simulink model "Closedloop"  (R2015b)
settings: Solver=ode4  StartTime=0.0  StopTime=600  FixedStep=DT  MaxStep=DT  RelTol=1e-3
values from neighbouring files (symbols this model uses):
  A1 = 1/Jr    (= 3.37837837838e-07)    [Run_closedloop.m]    (also in Run_img_closedloop.m)
  A2 = (Jr*(lambda-b31)-Cr)/Jr^2    [Run_closedloop.m]    (also in Run_img_closedloop.m)
  A3 = (Cr^2-a31*Jr-lambda*Cr*Jr)/Jr^2    [Run_closedloop.m]    (also in Run_img_closedloop.m)
  A4 = -a32/Jr    (= 0.00215037048063)    [Run_closedloop.m]    (also in Run_img_closedloop.m)
  A5 = (Cr-a33*Jr-lambda*Jr)/Jr^2    [Run_closedloop.m]    (also in Run_img_closedloop.m)
  b32 = Cls/ng/Jg    (= 21.4347948375)    [Run_closedloop.m]    (also in Run_img_closedloop.m)
  beta_opt = 2    [Run_closedloop.m]    (also in Run_img_closedloop.m)
  Cp = xlsread(filename)    [Run_closedloop.m]    (also in Run_img_closedloop.m)
  Cr = 625    [Run_closedloop.m]    (also in Run_img_closedloop.m)
  eta = 0.01    [Run_closedloop.m]    (also in Run_img_closedloop.m = 0.05)
  Jr = 2.96e6    (= 2960000)    [Run_closedloop.m]    (also in Run_img_closedloop.m)
  lambda = 0.1    [Run_closedloop.m]    (also in Run_img_closedloop.m = 10)
  lambda_opt = 7.1    [Run_closedloop.m]    (also in Run_img_closedloop.m)
  phi = 0.1    [Run_closedloop.m]    (also in Run_img_closedloop.m = 0.001)
  R = 35    [Run_closedloop.m]    (also in Run_img_closedloop.m)
  Rho = 1.225    [Run_closedloop.m]    (also in Run_img_closedloop.m)
undefined symbols (not defined in the file or in its folder): OutList, strmatch
settings Model: Creator=bjonkman  LastModifiedBy=alino
settings DataIOCC: SaveFormat=Array  SignalLoggingSaveFormat=ModelDataLogs  SaveOutput=off  SaveTime=off  SignalLoggingName=sigsOut
settings OptimizationCC: ExpressionDepthLimit=2147483647
settings DebuggingCC: SaveWithParameterizedLinksMsg=none  UnderspecifiedInitializationDetection=Classic  MergeDetectMultiDrivingBlocksExec=none  SignalResolutionControl=TryResolveAllWithWarning  MultiTaskDSMMsg=warning  MultiTaskCondExecSysMsg=none  FcnCallInpInsideContextMsg=EnableAllAsWarning  StateNameClashWarn=warning
settings HardwareCC: ProdBitPerPointer=32  ProdLargestAtomicFloat=None  ProdIntDivRoundTo=Undefined  ProdEndianess=Unspecified  ProdWordSize=32  ProdHWDeviceType=32-bit Generic  TargetUnknown=on
settings GRTTargetCC: GeneratePreprocessorConditionals=Disable all  CombineOutputUpdateFcns=off  GRTInterface=on
settings ConfigComp: CovModelRefEnable=Off

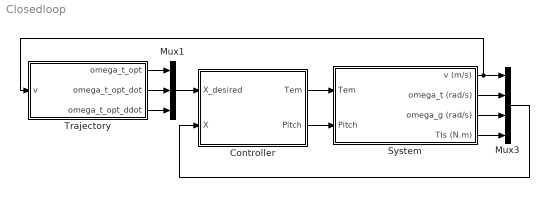
== system Closedloop ==
  Controller : Subsystem
  Mux1 : Mux  Inputs=3
  Mux3 : Mux
  System : Subsystem
  Trajectory : Subsystem
  wires:
  Mux3/1 -> Controller/2(X)
  Mux1/1 -> Controller/1(X_desired)
  Trajectory/2(omega_t_opt_dot) -> Mux1/2
  Trajectory/1(omega_t_opt) -> Mux1/1
  Controller/1(Tem) -> System/1(Tem)
  Controller/2(Pitch) -> System/2(Pitch)
  System/3(omega_g (rad/s)) -> Mux3/3
  System/4(Tls (N.m)) -> Mux3/4
  System/2(omega_t (rad/s)) -> Mux3/2
  System/1(v (m/s)) -> Mux3/1, Trajectory/1(v)
  Trajectory/3(omega_t_opt_ddot) -> Mux1/3

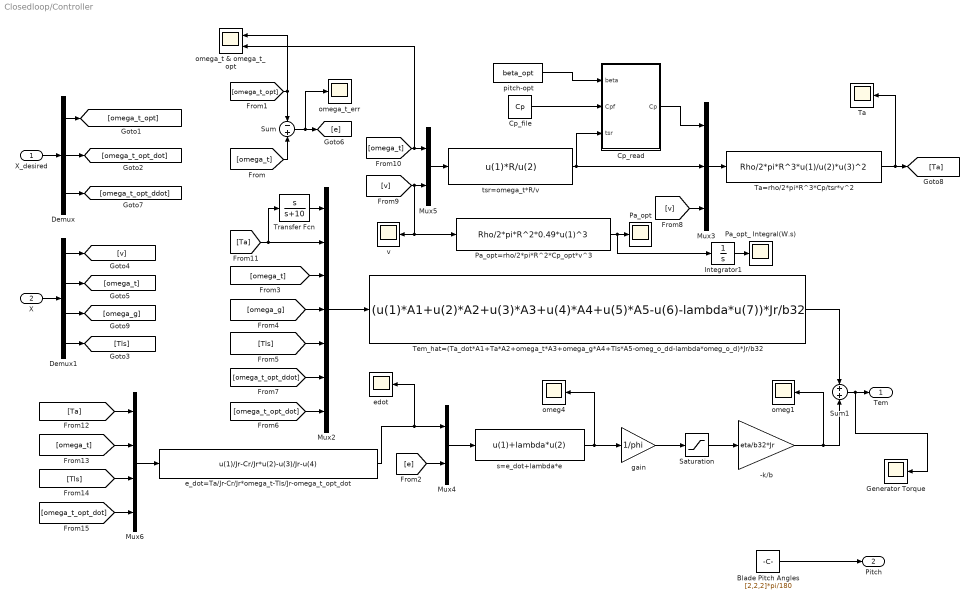
== system Closedloop/Controller ==
  X_desired : Inport
  X : Inport  Port=2
  -k/b : Gain  Gain=eta/b32*Jr
  Blade Pitch Angles : Constant  Value=[2,2,2]*pi/180
  Cp_file : Constant  Value=Cp
  Cp_read : MATLAB Function  TreatAsAtomicUnit=on
  Demux : Demux  Outputs=3
  Demux1 : Demux
  Generator Torque : Scope
  Integrator1 : Integrator
  Mux2 : Mux  Inputs=7
  Mux3 : Mux  Inputs=3
  Mux4 : Mux  Inputs=2
  Mux5 : Mux  Inputs=2
  Mux6 : Mux
  Pa_opt : Scope
  Pa_opt=rho/2*pi*R^2*Cp_opt*v^3 : Fcn  Expr=Rho/2*pi*R^2*0.49*u(1)^3
  Pa_opt_ Integral(W.s) : Scope
  Saturation : Saturate  UpperLimit=1  LowerLimit=-1
  Sum : Sum  Inputs=-+
  Sum1 : Sum  Inputs=+|+
  Ta : Scope
  Ta=rho/2*pi*R^3*Cp/tsr*v^2 : Fcn  Expr=Rho/2*pi*R^3*u(1)/u(2)*u(3)^2
  Tem_hat=(Ta_dot*A1+Ta*A2+omega_t*A3+omega_g*A4+Tls*A5-omeg_o_dd-lambda*omeg_o_d)*Jr/b32 : Fcn  Expr=(u(1)*A1+u(2)*A2+u(3)*A3+u(4)*A4+u(5)*A5-u(6)-lambda*u(7))*Jr/b32
  Transfer Fcn : TransferFcn  Numerator=[1 0]  Denominator=[1 10]
  e_dot=Ta/Jr-Cr/Jr*omega_t-Tls/Jr-omega_t_opt_dot : Fcn  Expr=u(1)/Jr-Cr/Jr*u(2)-u(3)/Jr-u(4)
  edot : Scope
  gain : Gain  Gain=1/phi
  omeg1 : Scope
  omeg4 : Scope
  omega_t & omega_t_opt : Scope  NumInputPorts=2
  omega_t_err : Scope
  pitch-opt : Constant  Value=beta_opt
  s=e_dot+lambda*e : Fcn  Expr=u(1)+lambda*u(2)
  tsr=omega_t*R/v : Fcn  Expr=u(1)*R/u(2)
  v : Scope
  Tem : Outport
  Pitch : Outport  Port=2
  wires:
  X_desired/1 -> Demux/1
  X/1 -> Demux1/1
  Tem_hat=(Ta_dot*A1+Ta*A2+omega_t*A3+omega_g*A4+Tls*A5-omeg_o_dd-lambda*omeg_o_d)*Jr/b32/1 -> Sum1/1
  Mux2/1 -> Tem_hat=(Ta_dot*A1+Ta*A2+omega_t*A3+omega_g*A4+Tls*A5-omeg_o_dd-lambda*omeg_o_d)*Jr/b32/1
  Mux4/1 -> s=e_dot+lambda*e/1
  s=e_dot+lambda*e/1 -> gain/1, omeg4/1
  [omega_t] -> Mux2/3
  Demux/1 -> [omega_t_opt]
  Demux/2 -> [omega_t_opt_dot]
  Demux1/1 -> [v]
  Demux1/2 -> [omega_t]
  Demux1/3 -> [omega_g]
  Blade Pitch Angles/1 -> Pitch/1
  Demux1/4 -> [Tls]
  Sum/1 -> omega_t_err/1, [e]
  [omega_t] -> Sum/2
  [omega_t_opt] -> omega_t & omega_t_opt/1, Sum/1
  [e] -> Mux4/2
  Demux/3 -> [omega_t_opt_ddot]
  [omega_g] -> Mux2/4
  [Tls] -> Mux2/5
  Mux3/1 -> Ta=rho/2*pi*R^3*Cp/tsr*v^2/1
  [v] -> Mux3/3
  Mux5/1 -> tsr=omega_t*R/v/1
  [v] -> Pa_opt=rho/2*pi*R^2*Cp_opt*v^3/1, v/1, Mux5/2
  [omega_t] -> omega_t & omega_t_opt/2, Mux5/1
  tsr=omega_t*R/v/1 -> Mux3/2, Cp_read/3(tsr)
  Ta=rho/2*pi*R^3*Cp/tsr*v^2/1 -> Ta/1, [Ta]
  [Ta] -> Transfer Fcn/1, Mux2/2
  Transfer Fcn/1 -> Mux2/1
  Mux6/1 -> e_dot=Ta/Jr-Cr/Jr*omega_t-Tls/Jr-omega_t_opt_dot/1
  e_dot=Ta/Jr-Cr/Jr*omega_t-Tls/Jr-omega_t_opt_dot/1 -> edot/1, Mux4/1
  [Ta] -> Mux6/1
  [omega_t] -> Mux6/2
  [Tls] -> Mux6/3
  [omega_t_opt_dot] -> Mux6/4
  Cp_read/1(Cp) -> Mux3/1
  Cp_file/1 -> Cp_read/2(Cpf)
  pitch-opt/1 -> Cp_read/1(beta)
  Sum1/1 -> Generator Torque/1, Tem/1
  [omega_t_opt_dot] -> Mux2/7
  [omega_t_opt_ddot] -> Mux2/6
  Saturation/1 -> -k/b/1
  gain/1 -> Saturation/1
  -k/b/1 -> omeg1/1, Sum1/2
  Pa_opt=rho/2*pi*R^2*Cp_opt*v^3/1 -> Integrator1/1, Pa_opt/1
  Integrator1/1 -> Pa_opt_ Integral(W.s)/1

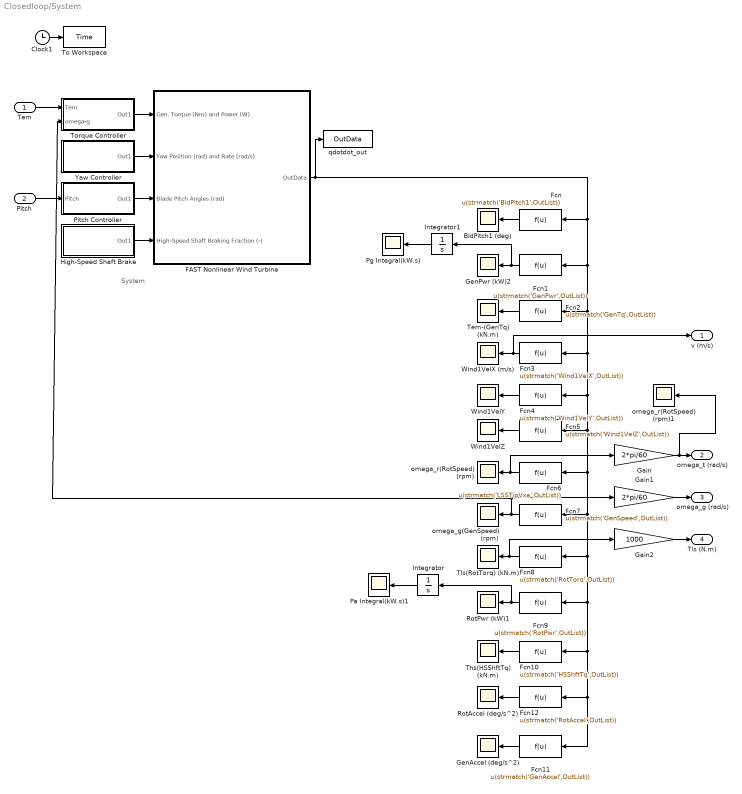
== system Closedloop/System ==
  note: System
  Tem : Inport
  Pitch : Inport  Port=2
  BldPitch1 (deg) : Scope
  Clock1 : Clock
  FAST Nonlinear Wind Turbine : Subsystem  mask(FAST Nonlinear Wind Turbine){}
      mask help: This block contains the FAST S-Function.
      mask init:
      | clear FAST_SFunc
  Fcn : Fcn  Expr=u(strmatch('BldPitch1',OutList))
  Fcn1 : Fcn  Expr=u(strmatch('GenPwr',OutList))
  Fcn10 : Fcn  Expr=u(strmatch('HSShftTq',OutList))
  Fcn11 : Fcn  Expr=u(strmatch('GenAccel',OutList))
  Fcn12 : Fcn  Expr=u(strmatch('RotAccel',OutList))
  Fcn2 : Fcn  Expr=u(strmatch('GenTq',OutList))
  Fcn3 : Fcn  Expr=u(strmatch('Wind1VelX',OutList))
  Fcn4 : Fcn  Expr=u(strmatch('Wind1VelY',OutList))
  Fcn5 : Fcn  Expr=u(strmatch('Wind1VelZ',OutList))
  Fcn6 : Fcn  Expr=u(strmatch('LSSTipVxa',OutList))
  Fcn7 : Fcn  Expr=u(strmatch('GenSpeed',OutList))
  Fcn8 : Fcn  Expr=u(strmatch('RotTorq',OutList))
  Fcn9 : Fcn  Expr=u(strmatch('RotPwr',OutList))
  Gain : Gain  Gain=2*pi/60
  Gain1 : Gain  Gain=2*pi/60
  Gain2 : Gain  Gain=1000
  GenAccel (deg/s^2) : Scope
  GenPwr (kW)2 : Scope
  High-Speed Shaft Brake : Subsystem
  Integrator : Integrator
  Integrator1 : Integrator
  Pa Integral(kW.s)1 : Scope
  Pg Integral(kW.s) : Scope
  Pitch Controller : Subsystem
  RotAccel (deg/s^2) : Scope
  RotPwr (kW)1 : Scope
  Tem-(GenTq) (kN.m) : Scope
  Ths(HSShftTq) (kN.m) : Scope
  Tls(RotTorq) (kN.m) : Scope
  To Workspace : ToWorkspace  VariableName=Time  SampleTime=-1
  Torque Controller : Subsystem
  Wind1VelX (m/s) : Scope
  Wind1VelY : Scope
  Wind1VelZ : Scope
  Yaw Controller : Subsystem
  omega_g(GenSpeed) (rpm) : Scope
  omega_r(RotSpeed) (rpm) : Scope
  omega_r(RotSpeed) (rpm)1 : Scope
  qdotdot_out : ToWorkspace  VariableName=OutData  SampleTime=-1
  v (m/s) : Outport
  omega_t (rad/s) : Outport  Port=2
  omega_g (rad/s) : Outport  Port=3
  Tls (N.m) : Outport  Port=4
  wires:
  Clock1/1 -> To Workspace/1
  Torque Controller/1(Out1) -> FAST Nonlinear Wind Turbine/1(Gen. Torque (Nm) and Power (W))
  Yaw Controller/1(Out1) -> FAST Nonlinear Wind Turbine/2(Yaw Position (rad) and Rate (rad/s))
  Pitch Controller/1(Out1) -> FAST Nonlinear Wind Turbine/3(Blade Pitch Angles (rad))
  High-Speed Shaft Brake/1(Out1) -> FAST Nonlinear Wind Turbine/4(High-Speed Shaft Braking Fraction (-))
  Fcn/1 -> BldPitch1 (deg)/1
  Fcn2/1 -> Tem-(GenTq) (kN.m)/1
  Fcn3/1 -> v (m/s)/1, Wind1VelX (m/s)/1
  Fcn4/1 -> Wind1VelY/1
  Fcn5/1 -> Wind1VelZ/1
  Fcn6/1 -> Gain/1, omega_r(RotSpeed) (rpm)/1
  Fcn7/1 -> Torque Controller/2(omega-g), Gain1/1, omega_g(GenSpeed) (rpm)/1
  Fcn8/1 -> Gain2/1, Tls(RotTorq) (kN.m)/1
  Fcn9/1 -> RotPwr (kW)1/1, Integrator/1
  Fcn10/1 -> Ths(HSShftTq) (kN.m)/1
  Fcn12/1 -> RotAccel (deg/s^2)/1
  FAST Nonlinear Wind Turbine/1(OutData) -> Fcn11/1, Fcn12/1, Fcn10/1, Fcn9/1, Fcn8/1, Fcn7/1, Fcn6/1, Fcn5/1, Fcn4/1, Fcn3/1, Fcn2/1, Fcn1/1, Fcn/1, qdotdot_out/1
  Fcn11/1 -> GenAccel (deg/s^2)/1
  Tem/1 -> Torque Controller/1(Tem)
  Gain/1 -> omega_r(RotSpeed) (rpm)1/1, omega_t (rad/s)/1
  Gain1/1 -> omega_g (rad/s)/1
  Gain2/1 -> Tls (N.m)/1
  Pitch/1 -> Pitch Controller/1(Pitch)
  Integrator/1 -> Pa Integral(kW.s)1/1
  Fcn1/1 -> GenPwr (kW)2/1, Integrator1/1
  Integrator1/1 -> Pg Integral(kW.s)/1

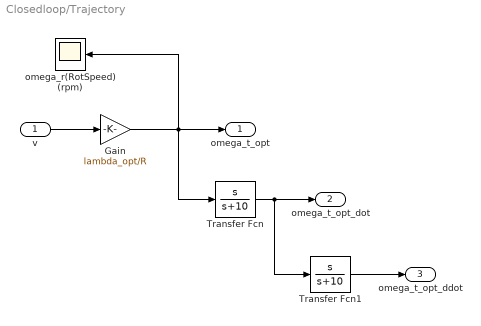
== system Closedloop/Trajectory ==
  v : Inport
  Gain : Gain  Gain=lambda_opt/R
  Transfer Fcn : TransferFcn  Numerator=[1 0]  Denominator=[1 10]
  Transfer Fcn1 : TransferFcn  Numerator=[1 0]  Denominator=[1 10]
  omega_r(RotSpeed) (rpm) : Scope
  omega_t_opt : Outport
  omega_t_opt_dot : Outport  Port=2
  omega_t_opt_ddot : Outport  Port=3
  wires:
  Transfer Fcn/1 -> Transfer Fcn1/1, omega_t_opt_dot/1
  v/1 -> Gain/1
  Gain/1 -> omega_r(RotSpeed) (rpm)/1, Transfer Fcn/1, omega_t_opt/1
  Transfer Fcn1/1 -> omega_t_opt_ddot/1

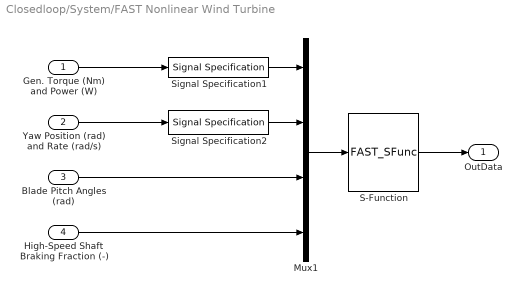
== system Closedloop/System/FAST Nonlinear Wind Turbine ==
  Gen. Torque (Nm) and Power (W) : Inport
  Yaw Position (rad) and Rate (rad/s) : Inport  Port=2
  Blade Pitch Angles (rad) : Inport  Port=3
  High-Speed Shaft Braking Fraction (-) : Inport  Port=4
  Mux1 : Mux
  S-Function : S-Function  FunctionName=FAST_SFunc  Parameters=FAST_InputFileName, TMax, 0  SFunctionDeploymentMode=off  EnableBusSupport=off
  Signal Specification1 : SignalSpecification  OutDataTypeStr=double  Dimensions=2
  Signal Specification2 : SignalSpecification  OutDataTypeStr=double  Dimensions=2
  OutData : Outport
  wires:
  Gen. Torque (Nm) and Power (W)/1 -> Signal Specification1/1
  S-Function/1 -> OutData/1
  Mux1/1 -> S-Function/1
  Blade Pitch Angles (rad)/1 -> Mux1/3
  Yaw Position (rad) and Rate (rad/s)/1 -> Signal Specification2/1
  Signal Specification1/1 -> Mux1/1
  Signal Specification2/1 -> Mux1/2
  High-Speed Shaft Braking Fraction (-)/1 -> Mux1/4

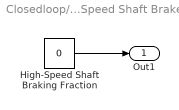
== system Closedloop/System/High-Speed Shaft Brake ==
  High-Speed Shaft Braking Fraction : Constant  Value=0
  Out1 : Outport
  wires:
  High-Speed Shaft Braking Fraction/1 -> Out1/1

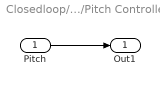
== system Closedloop/System/Pitch Controller ==
  Pitch : Inport
  Out1 : Outport
  wires:
  Pitch/1 -> Out1/1

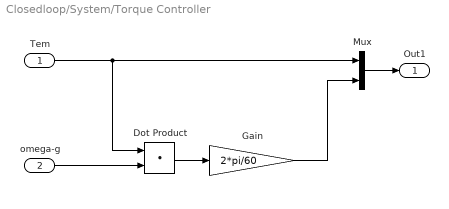
== system Closedloop/System/Torque Controller ==
  Tem : Inport
  omega-g : Inport  Port=2
  Dot Product : DotProduct  InputSameDT=on  OutDataTypeStr=Inherit: Inherit via internal rule
  Gain : Gain  Gain=2*pi/60
  Mux : Mux  Inputs=2
  Out1 : Outport
  wires:
  Mux/1 -> Out1/1
  Tem/1 -> Dot Product/1, Mux/1
  omega-g/1 -> Dot Product/2
  Dot Product/1 -> Gain/1
  Gain/1 -> Mux/2

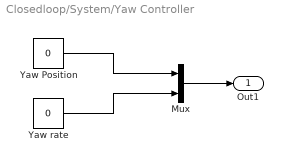
== system Closedloop/System/Yaw Controller ==
  Mux : Mux  Inputs=2
  Yaw Position : Constant  Value=0
  Yaw rate : Constant  Value=0
  Out1 : Outport
  wires:
  Mux/1 -> Out1/1
  Yaw Position/1 -> Mux/1
  Yaw rate/1 -> Mux/2

== matlab function Closedloop/Controller/Cp_read ==
  data: beta input; Cpf input; Cp output; tsr input
function Cp = fcn(beta,Cpf,tsr)

    if (tsr>19 || beta>90) 
        Cp=0;
    else
    beta1=floor(beta)+1;
    tsr1=floor(tsr*10);
    beta2=beta1+1;
    tsr2=tsr1+1;
    betap=beta-floor(beta);
    tsrp=tsr*10-floor(tsr*10);
    Cp1=Cpf(beta1,tsr1)+betap*(Cpf(beta2,tsr1)-Cpf(beta1,tsr1));
    Cp2=Cpf(beta1,tsr2)+betap*(Cpf(beta2,tsr2)-Cpf(beta1,tsr2));
    Cp=tsrp*(Cp2-Cp1)+Cp1;
    end
end
